simulink model "Auxiliary_Models"  (R2020b)
settings: Solver=VariableStepAuto  StartTime=0.0  StopTime=10.0  RelTol=1e-3
undefined symbols (not defined in the file or in its folder): Actuators, Ki, Klp, Klz, Kp, Kr, TestSequence, TrimPoint
libraries: simulink x19
settings Model: Creator=NicolasS  LastModifiedBy=benjaminh

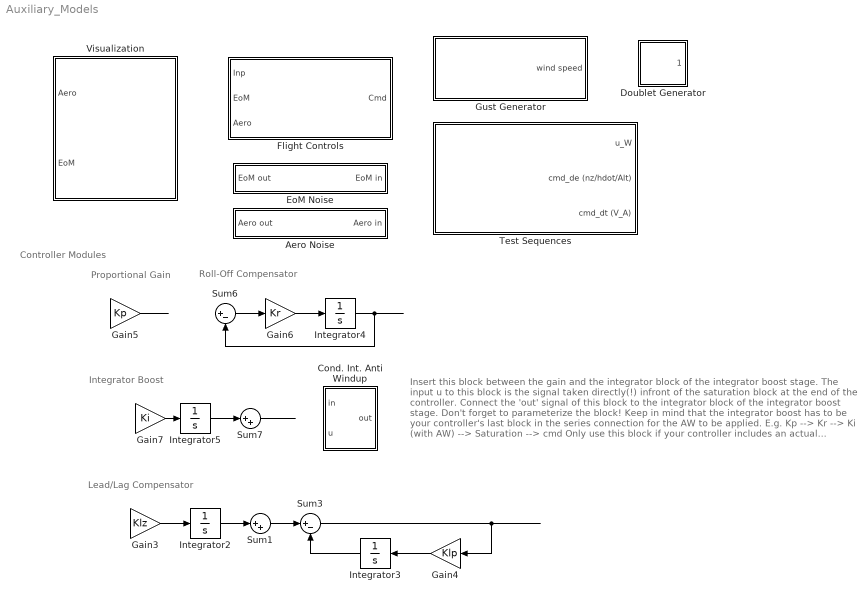
== system Auxiliary_Models ==
  note: Insert this block between the gain and the integrator block of the integrator boost stage.
      | The input u to this block is the signal taken directly(!) infront of the saturation block at the end of the controller. Connect the 'out' signal of this block to the integrator block of the integrator boost stage. Don't forget to parameterize the block!
      | Keep in mind that the integrator boost has to be your controller's last block in the series connection for the AW to be applied. E.g. Kp --> Kr --> Ki (with AW) --> Saturation --> cmd
      | Only use this block if your controller includes an actual integrator (integrator boost/pole at zero).
  note: Controller Modules
  note: Integrator Boost
  note: Roll-Off Compensator
  note: Proportional
      | Gain
  note: Lead/Lag Compensator
  Aero Noise : Subsystem
  Cond. Int. Anti Windup : Subsystem  mask(Integrator Anti-Windup){max_u=inf, min_u=-inf, negative_sign=off}
      mask prompts: max_u "Maximum control signal"; min_u "Minimum control signal"; negative_sign "Negative amplification in control law"
      mask help:
      | This block provides integration using the "conditional integration" anti-windup compensation.
      | It compares the sign of the error and the sign of the control signal and stops integration in case the error drives saturation.
      mask Help:
      | This block provides integration using the "conditional integration" anti-windup compensation. It stops or continues integration depending on the sign of the integrator input (control error) and the commanded control signal. Only if the input would further increase the already saturated integrator output, integration is stopped. This method is different from "integrator clamping" and and "integrator back calculation" and usually provides better recovery properties.
      | 
      | In a standard control architecture the inputs are as follows:
      | INPUT is the error signal r-y
      | RESET is a reset signal. The integrator state is reseted on either rising or falling edges
      | X0 is the initial condition for the integrator
      | U is the commanded control signal
      | 
      | For the anti-windup to work as intended, a saturation block must be placed on the ouput of the control command being fed to the associated actuator, which should include all control signal contributions (e.g. from proportional feedback and inner loops). U is the signal before this saturation.
      | 
      | The default logic assumes a plant with positive steady-state gain to be controlled. This translates to the following logic:
      | For commanded control signal u, saturation limits Umax and Umin, and error e,
      | If u is in bounds, do nothing
      | If u >= Umax AND e > 0, stop integrating
      | If u >= Umax AND e < 0, continue integrating
      | If u <= Umin AND e > 0, continue integrating
      | If u <= Umin AND e < 0, stop integrating
      | 
      | If a plant with negative steady-state gain is to be controlled (e.g. pitch), the windup logic may changed using the NEGATIVE SIGN option. (Note: If unsure check if the controller gains are negative. If yes, check the NEGATIVE SIGN option)
      | This then translates to the logic:
      | If u is in bounds, do nothing
      | If u >= Umax AND e < 0, stop integrating
      | If u >= Umax AND e > 0, continue integrating
      | If u <= Umin AND e < 0, continue integrating
      | If u <= Umin AND e > 0, stop integrating
  Doublet Generator : Subsystem  mask(DoubletGenerator){timeon=0, pulsewidth=1, amplitude=1}
      mask prompts: timeon "Time Start"; pulsewidth "Pulse Duration"
      mask help:
      | Doublet Generator.
      | Ouputs doublet of specificed amplitude and duration.
      |
      | If start/duration/amplitude parameters are vectors, then output is multichannel.
      mask Display: plot([.1 .3 .3001 .4 .4001 .5  .5001 .7],[0 0 1 1 -1 -1 0 0])
  EoM Noise : Subsystem
  Flight Controls : Subsystem
  Gain3 : Gain  Gain=Klz
  Gain4 : Gain  Gain=Klp
  Gain5 : Gain  Gain=Kp
  Gain6 : Gain  Gain=Kr
  Gain7 : Gain  Gain=Ki
  Gust Generator : Subsystem  mask{gust_start=0, gust_duration=0, gust_amplitude=0}
      mask prompts: gust_start "start time of the gust in sec"; gust_duration "gust duration in sec"; gust_amplitude "maximum gust speed in m/s"
      mask DialogControl ParameterGroupVar Prompt: gust characteristics
  Integrator{2..5} (4 alike) : Integrator  UpperSaturationLimit=max(Actuators.Limits.u_max_He)  LowerSaturationLimit=min(Actuators.Limits.u_max_He)  ContinuousStateAttributes='K'
  Sum1 : Sum  Inputs=|++
  Sum3 : Sum  Inputs=|+-
  Sum6 : Sum  Inputs=|+-
  Sum7 : Sum  Inputs=|++
  Test Sequences : Subsystem  InitFcn=|  StopFcn=clear TestSequence
      | if not(exist('TestSequence','var'))
      |        TestSequence = 0;
      | end
  Visualization : Subsystem
  wires:
  Sum7/1 -> ?
  Gain7/1 -> Integrator5/1
  Sum6/1 -> Gain6/1
  Integrator5/1 -> Sum7/1
  Gain6/1 -> Integrator4/1
  ? -> Gain5/1
  ? -> Gain7/1, Sum7/2
  Gain5/1 -> ?
  ? -> Sum6/1
  Integrator4/1 -> Sum6/2
  ? -> Sum1/2, Gain3/1
  Integrator2/1 -> Sum1/1
  Sum1/1 -> Sum3/1
  Gain4/1 -> Integrator3/1
  Integrator3/1 -> Sum3/2
  Sum3/1 -> Gain4/1
  Gain3/1 -> Integrator2/1

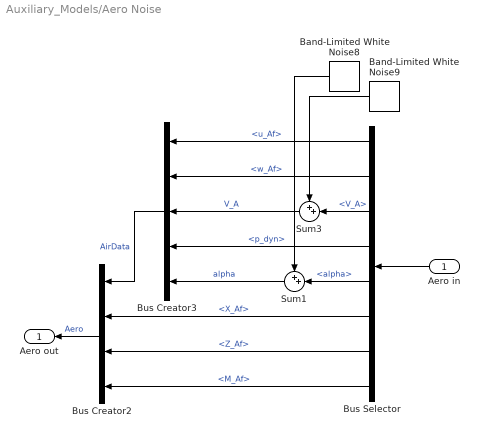
== system Auxiliary_Models/Aero Noise ==
  Aero in : Inport  OutDataTypeStr=Bus: Aero
  Band-Limited White Noise8 : simulink/Sources/Band-Limited White Noise  Cov=1E-7  Ts=0.01  seed=3324
  Band-Limited White Noise9 : simulink/Sources/Band-Limited White Noise  Cov=1E-3  Ts=0.05  seed=8153
  Bus Creator2 : BusCreator  Inputs=4  OutDataTypeStr=Bus: Aero
  Bus Creator3 : BusCreator  Inputs=5  OutDataTypeStr=Bus: AirData
  Bus Selector : BusSelector  OutputSignals=AirData.u_Af,AirData.w_Af,AirData.V_A,AirData.p_dyn,AirData.alpha,X_Af,Z_Af,M_Af
  Sum1 : Sum  Inputs=++|
  Sum3 : Sum  Inputs=++|
  Aero out : Outport  OutDataTypeStr=Bus: Aero
  wires:
  Aero in/1 -> Bus Selector/1
  Bus Creator3/1 -> Bus Creator2/1  "AirData"
  Bus Selector/6 -> Bus Creator2/2  "<X_Af>"
  Bus Selector/7 -> Bus Creator2/3  "<Z_Af>"
  Bus Selector/8 -> Bus Creator2/4  "<M_Af>"
  Bus Creator2/1 -> Aero out/1  "Aero"
  Bus Selector/1 -> Bus Creator3/1  "<u_Af>"
  Bus Selector/2 -> Bus Creator3/2  "<w_Af>"
  Bus Selector/3 -> Sum3/2  "<V_A>"
  Bus Selector/5 -> Sum1/2  "<alpha>"
  Band-Limited White Noise8/1 -> Sum1/1
  Sum1/1 -> Bus Creator3/5  "alpha"
  Bus Selector/4 -> Bus Creator3/4  "<p_dyn>"
  Band-Limited White Noise9/1 -> Sum3/1
  Sum3/1 -> Bus Creator3/3  "V_A"

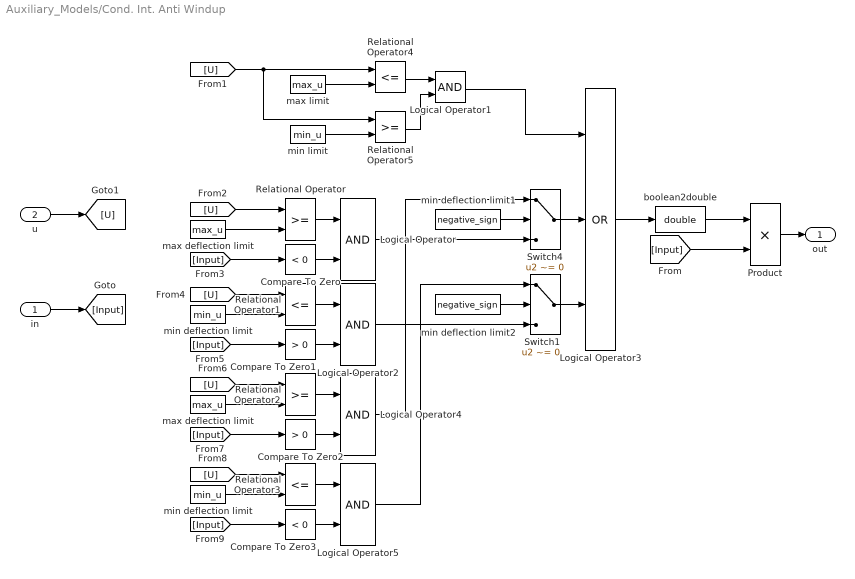
== system Auxiliary_Models/Cond. Int. Anti Windup ==
  in : Inport
  u : Inport  Port=2
  Compare To Zero : simulink/Logic and Bit Operations/Compare To Zero  relop=<  OutDataTypeStr=uint8
  Compare To Zero1 : simulink/Logic and Bit Operations/Compare To Zero  relop=>  OutDataTypeStr=uint8
  Compare To Zero2 : simulink/Logic and Bit Operations/Compare To Zero  relop=>  OutDataTypeStr=uint8
  Compare To Zero3 : simulink/Logic and Bit Operations/Compare To Zero  relop=<  OutDataTypeStr=uint8
  Logical Operator{,1..2,4..5} (5 alike) : Logic  AllPortsSameDT=off  OutDataTypeStr=boolean
  Logical Operator3 : Logic  Operator=OR  Inputs=3  AllPortsSameDT=off  OutDataTypeStr=boolean
  Product : Product
  Relational Operator : RelationalOperator  OutDataTypeStr=boolean  RndMeth=Nearest
  Relational Operator1 : RelationalOperator  Operator=<=  OutDataTypeStr=boolean  RndMeth=Nearest
  Relational Operator2 : RelationalOperator  OutDataTypeStr=boolean  RndMeth=Nearest
  Relational Operator3 : RelationalOperator  Operator=<=  OutDataTypeStr=boolean  RndMeth=Nearest
  Relational Operator4 : RelationalOperator  Operator=<=  OutDataTypeStr=boolean  RndMeth=Nearest
  Relational Operator5 : RelationalOperator  OutDataTypeStr=boolean  RndMeth=Nearest
  Switch1 : Switch  Criteria=u2 ~= 0
  Switch4 : Switch  Criteria=u2 ~= 0
  boolean2double : DataTypeConversion  OutDataTypeStr=double
  max deflection limit : Constant  Value=max_u  SampleTime=-1
  "max deflection limit " : Constant  Value=max_u  SampleTime=-1
  max limit : Constant  Value=max_u  SampleTime=-1
  min deflection limit : Constant  Value=min_u  SampleTime=-1
  "min deflection limit " : Constant  Value=min_u  SampleTime=-1
  min deflection limit1 : Constant  Value=negative_sign  SampleTime=-1
  min deflection limit2 : Constant  Value=negative_sign  SampleTime=-1
  min limit : Constant  Value=min_u  SampleTime=-1
  out : Outport
  wires:
  Product/1 -> out/1
  Logical Operator3/1 -> boolean2double/1
  boolean2double/1 -> Product/1
  [Input] -> Product/2
  [Input] -> Compare To Zero3/1
  [U] -> Relational Operator3/1
  [Input] -> Compare To Zero2/1
  [U] -> Relational Operator2/1
  [Input] -> Compare To Zero1/1
  [U] -> Relational Operator1/1
  [Input] -> Compare To Zero/1
  [U] -> Relational Operator/1
  [U] -> Relational Operator4/1, Relational Operator5/1
  u/1 -> [U]
  in/1 -> [Input]
  min limit/1 -> Relational Operator5/2
  Relational Operator5/1 -> Logical Operator1/2
  Relational Operator4/1 -> Logical Operator1/1
  max limit/1 -> Relational Operator4/2
  Logical Operator5/1 -> Switch1/1
  Logical Operator4/1 -> Switch4/1
  Logical Operator2/1 -> Switch1/3
  Logical Operator/1 -> Switch4/3
  min deflection limit1/1 -> Switch4/2
  Switch1/1 -> Logical Operator3/3
  min deflection limit2/1 -> Switch1/2
  max deflection limit/1 -> Relational Operator/2
  Compare To Zero/1 -> Logical Operator/2
  Relational Operator/1 -> Logical Operator/1
  Compare To Zero1/1 -> Logical Operator2/2
  Relational Operator1/1 -> Logical Operator2/1
  min deflection limit/1 -> Relational Operator1/2
  Switch4/1 -> Logical Operator3/2
  Logical Operator1/1 -> Logical Operator3/1
  Compare To Zero2/1 -> Logical Operator4/2
  Relational Operator2/1 -> Logical Operator4/1
  Compare To Zero3/1 -> Logical Operator5/2
  Relational Operator3/1 -> Logical Operator5/1
  "min deflection limit "/1 -> Relational Operator3/2
  "max deflection limit "/1 -> Relational Operator2/2

== system Auxiliary_Models/Doublet Generator ==
  Add : Sum  Inputs=+++
  DownStep : Step  Time=timeon+pulsewidth  After=-2  SampleTime=0
  Gain : Gain  Gain=amplitude
  UnStep : Step  Time=timeon+2*pulsewidth  SampleTime=0
  UpStep : Step  Time=timeon  SampleTime=0
  Doublet : Outport
  wires:
  UpStep/1 -> Add/1
  DownStep/1 -> Add/2
  UnStep/1 -> Add/3
  Add/1 -> Gain/1
  Gain/1 -> Doublet/1

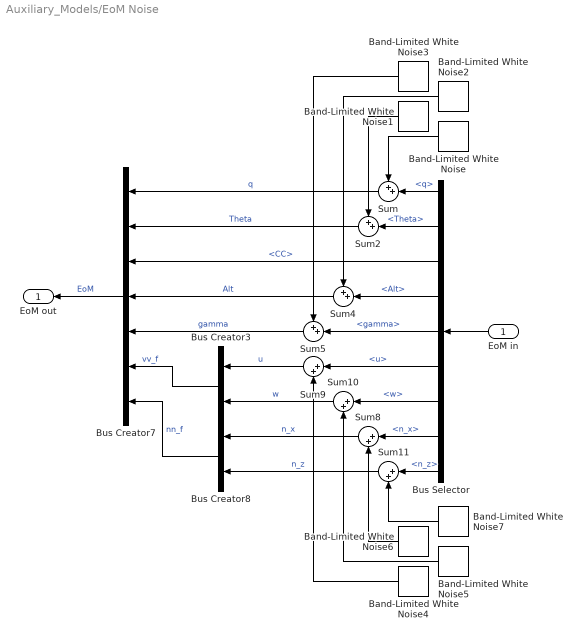
== system Auxiliary_Models/EoM Noise ==
  EoM in : Inport  OutDataTypeStr=Bus: EoM
  Band-Limited White Noise : simulink/Sources/Band-Limited White Noise  Cov=1E-5  Ts=0.01  seed=[23341]
  Band-Limited White Noise1 : simulink/Sources/Band-Limited White Noise  Cov=5E-7  Ts=0.01  seed=45875
  Band-Limited White Noise2 : simulink/Sources/Band-Limited White Noise  Cov=1E-4  Ts=0.1  seed=6874
  Band-Limited White Noise3 : simulink/Sources/Band-Limited White Noise  Cov=1E-7  Ts=0.01  seed=8153
  Band-Limited White Noise4 : simulink/Sources/Band-Limited White Noise  Cov=5E-5  Ts=0.1  seed=54769
  Band-Limited White Noise5 : simulink/Sources/Band-Limited White Noise  Cov=1E-4  Ts=0.01  seed=6932
  Band-Limited White Noise6 : simulink/Sources/Band-Limited White Noise  Cov=1E-5  Ts=0.01  seed=11452
  Band-Limited White Noise7 : simulink/Sources/Band-Limited White Noise  Cov=1E-5  Ts=0.01  seed=3324
  Bus Creator3 : BusCreator  Inputs=2  OutDataTypeStr=Bus: vv_f
  Bus Creator7 : BusCreator  Inputs=7  OutDataTypeStr=Bus: EoM
  Bus Creator8 : BusCreator  Inputs=2  OutDataTypeStr=Bus: nn_f
  Bus Selector : BusSelector  OutputSignals=q,Theta,CC,Alt,gamma,vv_f.u,vv_f.w,nn_f.n_x,nn_f.n_z
  Sum{,2,4..5} (4 alike) : Sum  Inputs=++|
  Sum{8..11} (4 alike) : Sum  Inputs=|++
  EoM out : Outport  OutDataTypeStr=Bus: EoM
  wires:
  Bus Selector/3 -> Bus Creator7/3  "<CC>"
  Bus Selector/9 -> Sum11/1  "<n_z>"
  Sum5/1 -> Bus Creator7/5  "gamma"
  Bus Creator8/1 -> Bus Creator7/7  "nn_f"
  Sum8/1 -> Bus Creator8/1  "n_x"
  Band-Limited White Noise/1 -> Sum/1
  Bus Selector/5 -> Sum5/2  "<gamma>"
  EoM in/1 -> Bus Selector/1
  Bus Selector/4 -> Sum4/2  "<Alt>"
  Bus Creator7/1 -> EoM out/1  "EoM"
  Band-Limited White Noise5/1 -> Sum10/2
  Bus Selector/8 -> Sum8/1  "<n_x>"
  Bus Creator3/1 -> Bus Creator7/6  "vv_f"
  Sum2/1 -> Bus Creator7/2  "Theta"
  Sum9/1 -> Bus Creator3/1  "u"
  Sum11/1 -> Bus Creator8/2  "n_z"
  Band-Limited White Noise3/1 -> Sum5/1
  Sum/1 -> Bus Creator7/1  "q"
  Band-Limited White Noise2/1 -> Sum4/1
  Bus Selector/6 -> Sum9/1  "<u>"
  Bus Selector/2 -> Sum2/2  "<Theta>"
  Band-Limited White Noise7/1 -> Sum11/2
  Bus Selector/7 -> Sum10/1  "<w>"
  Band-Limited White Noise4/1 -> Sum9/2
  Band-Limited White Noise1/1 -> Sum2/1
  Band-Limited White Noise6/1 -> Sum8/2
  Sum10/1 -> Bus Creator3/2  "w"
  Bus Selector/1 -> Sum/2  "<q>"
  Sum4/1 -> Bus Creator7/4  "Alt"

== system Auxiliary_Models/Flight Controls ==
  Inp : Inport
  EoM : Inport  Port=2  OutDataTypeStr=Bus: EoM
  Aero : Inport  Port=3  OutDataTypeStr=Bus: Aero
  Bus Creator2 : BusCreator  Inputs=2  OutDataTypeStr=Bus: Cmd
  Longitudinal Control Laws : Subsystem
  Cmd : Outport
  wires:
  EoM/1 -> Longitudinal Control Laws/2(EoM)
  Bus Creator2/1 -> Cmd/1  "Cmd"
  Longitudinal Control Laws/2(cmd_dt) -> Bus Creator2/2  "cmd_dt"
  Longitudinal Control Laws/1(cmd_de) -> Bus Creator2/1  "cmd_de"
  Inp/1 -> Longitudinal Control Laws/3(Inp)
  Aero/1 -> Longitudinal Control Laws/1(Aero)

== system Auxiliary_Models/Gust Generator ==
  1-cos gust : Subsystem  TreatAsAtomicUnit=on
  Clock : Clock
  Compare To Constant : simulink/Logic and Bit Operations/Compare To Constant  relop=>=  const=gust_start  OutDataTypeStr=boolean
  Constant : Constant  Value=0
  Sum : Sum  Inputs=+-|
  Switch : Switch  Criteria=u2 > Threshold  Threshold=gust_start+gust_duration
  time freeze : Subsystem  TreatAsAtomicUnit=on
  wind speed : Outport
  wires:
  time freeze/1(out) -> Sum/2
  Constant/1 -> Switch/1
  Clock/1 -> time freeze/1(in), Compare To Constant/1, Sum/1, Switch/2
  Compare To Constant/1 -> 1-cos gust/Enable, time freeze/Trigger
  Sum/1 -> 1-cos gust/1(in)
  1-cos gust/1(wind) -> Switch/3
  Switch/1 -> wind speed/1

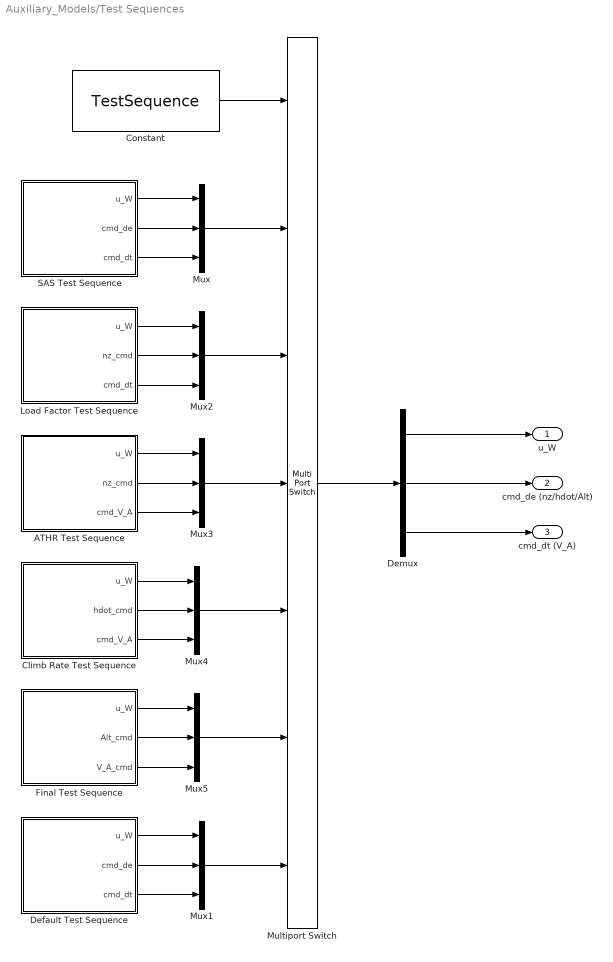
== system Auxiliary_Models/Test Sequences ==
  ATHR Test Sequence : Subsystem
  Climb Rate Test Sequence : Subsystem
  Constant : Constant  Value=TestSequence
  Default Test Sequence : Subsystem
  Demux : Demux  Outputs=3
  Final Test Sequence : Subsystem
  Load Factor Test Sequence : Subsystem
  Multiport Switch : MultiPortSwitch  Inputs=6
  Mux{,1..5} (6 alike) : Mux  Inputs=3
  SAS Test Sequence : Subsystem
  u_W : Outport
  cmd_de (nz/hdot/Alt) : Outport  Port=2
  cmd_dt (V_A) : Outport  Port=3
  wires:
  Demux/1 -> u_W/1
  Demux/2 -> cmd_de (nz/hdot/Alt)/1
  Demux/3 -> cmd_dt (V_A)/1
  Constant/1 -> Multiport Switch/1
  SAS Test Sequence/1(u_W) -> Mux/1
  SAS Test Sequence/2(cmd_de) -> Mux/2
  SAS Test Sequence/3(cmd_dt) -> Mux/3
  Mux/1 -> Multiport Switch/2
  Multiport Switch/1 -> Demux/1
  Default Test Sequence/1(u_W) -> Mux1/1
  Default Test Sequence/2(cmd_de) -> Mux1/2
  Default Test Sequence/3(cmd_dt) -> Mux1/3
  Mux1/1 -> Multiport Switch/7
  Load Factor Test Sequence/1(u_W) -> Mux2/1
  Load Factor Test Sequence/2(nz_cmd) -> Mux2/2
  Load Factor Test Sequence/3(cmd_dt) -> Mux2/3
  Mux2/1 -> Multiport Switch/3
  ATHR Test Sequence/1(u_W) -> Mux3/1
  ATHR Test Sequence/2(nz_cmd) -> Mux3/2
  ATHR Test Sequence/3(cmd_V_A) -> Mux3/3
  Mux3/1 -> Multiport Switch/4
  Climb Rate Test Sequence/1(u_W) -> Mux4/1
  Climb Rate Test Sequence/2(hdot_cmd) -> Mux4/2
  Climb Rate Test Sequence/3(cmd_V_A) -> Mux4/3
  Mux4/1 -> Multiport Switch/5
  Final Test Sequence/1(u_W) -> Mux5/1
  Final Test Sequence/2(Alt_cmd) -> Mux5/2
  Final Test Sequence/3(V_A_cmd) -> Mux5/3
  Mux5/1 -> Multiport Switch/6

== system Auxiliary_Models/Visualization ==
  Aero : Inport  OutDataTypeStr=Bus: Aero
  EoM : Inport  Port=2  OutDataTypeStr=Bus: EoM
  Bus Selector2 : BusSelector  OutputSignals=OOmega_f.q,vv_f.u,vv_f.w,PPhi.Theta,Position.Alt,nn_f.n_z
  Bus Selector3 : BusSelector  OutputSignals=AirData.alpha
  Gain11 : Gain  Gain=180/pi
  Gain8 : Gain  Gain=180/pi
  Gain9 : Gain  Gain=180/pi
  Scope2 : Scope  NumInputPorts=7
  wires:
  Gain8/1 -> Scope2/2  "q"
  Gain11/1 -> Scope2/1  "alpha"
  Gain9/1 -> Scope2/5  "Theta"
  Aero/1 -> Bus Selector3/1
  Bus Selector2/2 -> Scope2/3  "<u>"
  Bus Selector2/1 -> Gain8/1  "<q>"
  EoM/1 -> Bus Selector2/1
  Bus Selector2/6 -> Scope2/7  "<n_z>"
  Bus Selector2/5 -> Scope2/6  "<Alt>"
  Bus Selector3/1 -> Gain11/1  "<alpha>"
  Bus Selector2/3 -> Scope2/4  "<w>"
  Bus Selector2/4 -> Gain9/1  "<Theta>"

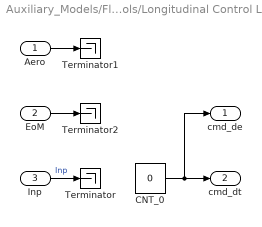
== system Auxiliary_Models/Flight Controls/Longitudinal Control Laws ==
  Aero : Inport  OutDataTypeStr=Bus: Aero
  EoM : Inport  Port=2  OutDataTypeStr=Bus: EoM
  Inp : Inport  Port=3
  CNT_0 : Constant  Value=0
  Terminator : Terminator
  Terminator1 : Terminator
  Terminator2 : Terminator
  cmd_de : Outport
  cmd_dt : Outport  Port=2
  wires:
  CNT_0/1 -> cmd_de/1, cmd_dt/1
  Inp/1 -> Terminator/1  "Inp"
  Aero/1 -> Terminator1/1
  EoM/1 -> Terminator2/1

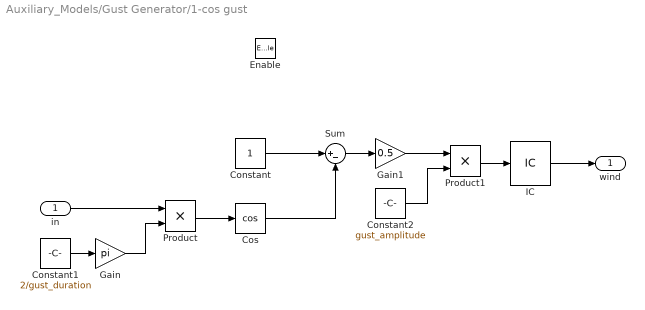
== system Auxiliary_Models/Gust Generator/1-cos gust ==
  in : Inport
  Enable : EnablePort  StatesWhenEnabling=reset
  Constant : Constant
  Constant1 : Constant  Value=2/gust_duration
  Constant2 : Constant  Value=gust_amplitude
  Cos : Trigonometry  Operator=cos
  Gain : Gain  Gain=pi
  Gain1 : Gain  Gain=0.5
  IC : InitialCondition  Value=0
  Product : Product
  Product1 : Product
  Sum : Sum  Inputs=|+-
  wind : Outport
  wires:
  IC/1 -> wind/1
  Constant1/1 -> Gain/1
  Product1/1 -> IC/1
  Product/1 -> Cos/1
  Cos/1 -> Sum/2
  Constant/1 -> Sum/1
  Gain/1 -> Product/2
  Gain1/1 -> Product1/1
  Sum/1 -> Gain1/1
  Constant2/1 -> Product1/2
  in/1 -> Product/1

== system Auxiliary_Models/Gust Generator/time freeze ==
  in : Inport
  Trigger : TriggerPort  VariantControl=Variant
  out : Outport  InitialOutput=0
  wires:
  in/1 -> out/1

== system Auxiliary_Models/Test Sequences/ATHR Test Sequence ==
  Add : Sum
  Constant1 : Constant  Value=0
  Constant2 : Constant  Value=sqrt(TrimPoint.States.ubar^2+TrimPoint.States.wbar^2)
  Doublet Generator : Subsystem  mask(DoubletGenerator){timeon=5, pulsewidth=30, amplitude=10}
      mask prompts: timeon "Time Start"; pulsewidth "Pulse Duration"
      mask help:
      | Doublet Generator.
      | Ouputs doublet of specificed amplitude and duration.
      |
      | If start/duration/amplitude parameters are vectors, then output is multichannel.
      mask Display: plot([.1 .3 .3001 .4 .4001 .5  .5001 .7],[0 0 1 1 -1 -1 0 0])
  Gust Generator : Subsystem  mask{gust_start=100, gust_duration=15, gust_amplitude=20}
      mask prompts: gust_start "start time of the gust in sec"; gust_duration "gust duration in sec"; gust_amplitude "maximum gust speed in m/s"
      mask DialogControl ParameterGroupVar Prompt: gust characteristics
  u_W : Outport  PortDimensions=1
  nz_cmd : Outport  Port=2
  cmd_V_A : Outport  Port=3
  wires:
  Constant1/1 -> nz_cmd/1  "nz_cmd"
  Doublet Generator/1(Doublet) -> Add/1
  Gust Generator/1(wind speed) -> u_W/1  "u_W"
  Add/1 -> cmd_V_A/1  "cmd_V_A"
  Constant2/1 -> Add/2  "nz_cmd"

== system Auxiliary_Models/Test Sequences/Climb Rate Test Sequence ==
  Constant1 : Constant  Value=0
  Constant2 : Constant  Value=sqrt(TrimPoint.States.ubar^2+TrimPoint.States.wbar^2)
  Doublet Generator : Subsystem  mask(DoubletGenerator){timeon=5, pulsewidth=20, amplitude=5}
      mask prompts: timeon "Time Start"; pulsewidth "Pulse Duration"
      mask help:
      | Doublet Generator.
      | Ouputs doublet of specificed amplitude and duration.
      |
      | If start/duration/amplitude parameters are vectors, then output is multichannel.
      mask Display: plot([.1 .3 .3001 .4 .4001 .5  .5001 .7],[0 0 1 1 -1 -1 0 0])
  u_W : Outport  PortDimensions=1
  hdot_cmd : Outport  Port=2
  cmd_V_A : Outport  Port=3
  wires:
  Doublet Generator/1(Doublet) -> hdot_cmd/1  "hdot_cmd"
  Constant1/1 -> u_W/1  "u_W"
  Constant2/1 -> cmd_V_A/1  "cmd_V_A"

== system Auxiliary_Models/Test Sequences/Default Test Sequence ==
  Constant : Constant  Value=TrimPoint.States.debar
  Constant1 : Constant  Value=0
  Constant2 : Constant  Value=TrimPoint.States.dtbar
  u_W : Outport  PortDimensions=1
  cmd_de : Outport  Port=2
  cmd_dt : Outport  Port=3
  wires:
  Constant/1 -> cmd_de/1  "cmd_de"
  Constant2/1 -> cmd_dt/1  "cmd_dt"
  Constant1/1 -> u_W/1  "u_W"

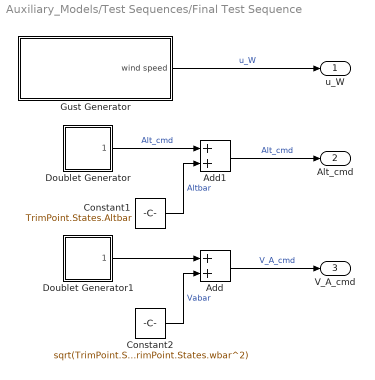
== system Auxiliary_Models/Test Sequences/Final Test Sequence ==
  Add : Sum
  Add1 : Sum
  Constant1 : Constant  Value=TrimPoint.States.Altbar
  Constant2 : Constant  Value=sqrt(TrimPoint.States.ubar^2+TrimPoint.States.wbar^2)
  Doublet Generator : Subsystem  mask(DoubletGenerator){timeon=5, pulsewidth=40, amplitude=100}
      mask prompts: timeon "Time Start"; pulsewidth "Pulse Duration"
      mask help:
      | Doublet Generator.
      | Ouputs doublet of specificed amplitude and duration.
      |
      | If start/duration/amplitude parameters are vectors, then output is multichannel.
      mask Display: plot([.1 .3 .3001 .4 .4001 .5  .5001 .7],[0 0 1 1 -1 -1 0 0])
  Doublet Generator1 : Subsystem  mask(DoubletGenerator){timeon=5, pulsewidth=60, amplitude=10}
      mask prompts: timeon "Time Start"; pulsewidth "Pulse Duration"
      mask help:
      | Doublet Generator.
      | Ouputs doublet of specificed amplitude and duration.
      |
      | If start/duration/amplitude parameters are vectors, then output is multichannel.
      mask Display: plot([.1 .3 .3001 .4 .4001 .5  .5001 .7],[0 0 1 1 -1 -1 0 0])
  Gust Generator : Subsystem  mask{gust_start=30, gust_duration=15, gust_amplitude=20}
      mask prompts: gust_start "start time of the gust in sec"; gust_duration "gust duration in sec"; gust_amplitude "maximum gust speed in m/s"
      mask DialogControl ParameterGroupVar Prompt: gust characteristics
  u_W : Outport  PortDimensions=1
  Alt_cmd : Outport  Port=2
  V_A_cmd : Outport  Port=3
  wires:
  Doublet Generator/1(Doublet) -> Add1/1  "Alt_cmd"
  Gust Generator/1(wind speed) -> u_W/1  "u_W"
  Add/1 -> V_A_cmd/1  "V_A_cmd"
  Doublet Generator1/1(Doublet) -> Add/1
  Constant2/1 -> Add/2  "Vabar"
  Constant1/1 -> Add1/2  "Altbar"
  Add1/1 -> Alt_cmd/1  "Alt_cmd"

== system Auxiliary_Models/Test Sequences/Load Factor Test Sequence ==
  Constant2 : Constant  Value=TrimPoint.States.dtbar
  Doublet Generator : Subsystem  mask(DoubletGenerator){timeon=5, pulsewidth=6, amplitude=0.2}
      mask prompts: timeon "Time Start"; pulsewidth "Pulse Duration"
      mask help:
      | Doublet Generator.
      | Ouputs doublet of specificed amplitude and duration.
      |
      | If start/duration/amplitude parameters are vectors, then output is multichannel.
      mask Display: plot([.1 .3 .3001 .4 .4001 .5  .5001 .7],[0 0 1 1 -1 -1 0 0])
  Gust Generator : Subsystem  mask{gust_start=20, gust_duration=15, gust_amplitude=20}
      mask prompts: gust_start "start time of the gust in sec"; gust_duration "gust duration in sec"; gust_amplitude "maximum gust speed in m/s"
      mask DialogControl ParameterGroupVar Prompt: gust characteristics
  u_W : Outport  PortDimensions=1
  nz_cmd : Outport  Port=2
  cmd_dt : Outport  Port=3
  wires:
  Doublet Generator/1(Doublet) -> nz_cmd/1  "nz_cmd"
  Constant2/1 -> cmd_dt/1  "cmd_dt"
  Gust Generator/1(wind speed) -> u_W/1  "u_W"

== system Auxiliary_Models/Test Sequences/SAS Test Sequence ==
  Constant2 : Constant  Value=TrimPoint.States.dtbar
  Gust Generator : Subsystem  mask{gust_start=15, gust_duration=15, gust_amplitude=20}
      mask prompts: gust_start "start time of the gust in sec"; gust_duration "gust duration in sec"; gust_amplitude "maximum gust speed in m/s"
      mask DialogControl ParameterGroupVar Prompt: gust characteristics
  Step : Step  Time=5  Before=TrimPoint.States.debar  After=TrimPoint.States.debar + deg2rad(-1)  SampleTime=0
  u_W : Outport  PortDimensions=1
  cmd_de : Outport  Port=2
  cmd_dt : Outport  Port=3
  wires:
  Step/1 -> cmd_de/1  "cmd_de"
  Constant2/1 -> cmd_dt/1  "cmd_dt"
  Gust Generator/1(wind speed) -> u_W/1  "u_W"

== system Auxiliary_Models/Test Sequences/ATHR Test Sequence/Doublet Generator ==
  Add : Sum  Inputs=+++
  DownStep : Step  Time=timeon+pulsewidth  After=-1  SampleTime=0
  Gain : Gain  Gain=amplitude
  UnStep : Step  Time=timeon+2*pulsewidth  After=-1  SampleTime=0
  UpStep : Step  Time=timeon  SampleTime=0
  Doublet : Outport
  wires:
  UpStep/1 -> Add/1
  DownStep/1 -> Add/2
  UnStep/1 -> Add/3
  Add/1 -> Gain/1
  Gain/1 -> Doublet/1

== system Auxiliary_Models/Test Sequences/ATHR Test Sequence/Gust Generator ==
  1-cos gust : Subsystem  TreatAsAtomicUnit=on
  Clock : Clock
  Compare To Constant : simulink/Logic and Bit Operations/Compare To Constant  relop=>=  const=gust_start  OutDataTypeStr=boolean
  Constant : Constant  Value=0
  Sum : Sum  Inputs=+-|
  Switch : Switch  Criteria=u2 > Threshold  Threshold=gust_start+gust_duration
  time freeze : Subsystem  TreatAsAtomicUnit=on
  wind speed : Outport
  wires:
  time freeze/1(out) -> Sum/2
  Constant/1 -> Switch/1
  Clock/1 -> time freeze/1(in), Compare To Constant/1, Sum/1, Switch/2
  Compare To Constant/1 -> 1-cos gust/Enable, time freeze/Trigger
  Sum/1 -> 1-cos gust/1(in)
  1-cos gust/1(wind) -> Switch/3
  Switch/1 -> wind speed/1

== system Auxiliary_Models/Test Sequences/Climb Rate Test Sequence/Doublet Generator ==
  Add : Sum  Inputs=+++
  DownStep : Step  Time=timeon+pulsewidth  After=-2  SampleTime=0
  Gain : Gain  Gain=amplitude
  UnStep : Step  Time=timeon+2*pulsewidth  SampleTime=0
  UpStep : Step  Time=timeon  SampleTime=0
  Doublet : Outport
  wires:
  UpStep/1 -> Add/1
  DownStep/1 -> Add/2
  UnStep/1 -> Add/3
  Add/1 -> Gain/1
  Gain/1 -> Doublet/1

== system Auxiliary_Models/Test Sequences/Final Test Sequence/Doublet Generator ==
  Add : Sum  Inputs=+++
  DownStep : Step  Time=timeon+pulsewidth  After=-2  SampleTime=0
  Gain : Gain  Gain=amplitude
  UnStep : Step  Time=timeon+2*pulsewidth  SampleTime=0
  UpStep : Step  Time=timeon  SampleTime=0
  Doublet : Outport
  wires:
  UpStep/1 -> Add/1
  DownStep/1 -> Add/2
  UnStep/1 -> Add/3
  Add/1 -> Gain/1
  Gain/1 -> Doublet/1

== system Auxiliary_Models/Test Sequences/Final Test Sequence/Doublet Generator1 ==
  Add : Sum  Inputs=+++
  DownStep : Step  Time=timeon+pulsewidth  SampleTime=0
  Gain : Gain  Gain=amplitude
  UnStep : Step  Time=timeon+2*pulsewidth  After=-1  SampleTime=0
  UpStep : Step  Time=timeon  SampleTime=0
  Doublet : Outport
  wires:
  UpStep/1 -> Add/1
  DownStep/1 -> Add/2
  UnStep/1 -> Add/3
  Add/1 -> Gain/1
  Gain/1 -> Doublet/1

== system Auxiliary_Models/Test Sequences/Final Test Sequence/Gust Generator ==
  1-cos gust : Subsystem  TreatAsAtomicUnit=on
  Clock : Clock
  Compare To Constant : simulink/Logic and Bit Operations/Compare To Constant  relop=>=  const=gust_start  OutDataTypeStr=boolean
  Constant : Constant  Value=0
  Sum : Sum  Inputs=+-|
  Switch : Switch  Criteria=u2 > Threshold  Threshold=gust_start+gust_duration
  time freeze : Subsystem  TreatAsAtomicUnit=on
  wind speed : Outport
  wires:
  time freeze/1(out) -> Sum/2
  Constant/1 -> Switch/1
  Clock/1 -> time freeze/1(in), Compare To Constant/1, Sum/1, Switch/2
  Compare To Constant/1 -> 1-cos gust/Enable, time freeze/Trigger
  Sum/1 -> 1-cos gust/1(in)
  1-cos gust/1(wind) -> Switch/3
  Switch/1 -> wind speed/1

== system Auxiliary_Models/Test Sequences/Load Factor Test Sequence/Doublet Generator ==
  Add : Sum  Inputs=+++
  DownStep : Step  Time=timeon+pulsewidth  After=-2  SampleTime=0
  Gain : Gain  Gain=amplitude
  UnStep : Step  Time=timeon+2*pulsewidth  SampleTime=0
  UpStep : Step  Time=timeon  SampleTime=0
  Doublet : Outport
  wires:
  UpStep/1 -> Add/1
  DownStep/1 -> Add/2
  UnStep/1 -> Add/3
  Add/1 -> Gain/1
  Gain/1 -> Doublet/1

== system Auxiliary_Models/Test Sequences/Load Factor Test Sequence/Gust Generator ==
  1-cos gust : Subsystem  TreatAsAtomicUnit=on
  Clock : Clock
  Compare To Constant : simulink/Logic and Bit Operations/Compare To Constant  relop=>=  const=gust_start  OutDataTypeStr=boolean
  Constant : Constant  Value=0
  Sum : Sum  Inputs=+-|
  Switch : Switch  Criteria=u2 > Threshold  Threshold=gust_start+gust_duration
  time freeze : Subsystem  TreatAsAtomicUnit=on
  wind speed : Outport
  wires:
  time freeze/1(out) -> Sum/2
  Constant/1 -> Switch/1
  Clock/1 -> time freeze/1(in), Compare To Constant/1, Sum/1, Switch/2
  Compare To Constant/1 -> 1-cos gust/Enable, time freeze/Trigger
  Sum/1 -> 1-cos gust/1(in)
  1-cos gust/1(wind) -> Switch/3
  Switch/1 -> wind speed/1

== system Auxiliary_Models/Test Sequences/SAS Test Sequence/Gust Generator ==
  1-cos gust : Subsystem  TreatAsAtomicUnit=on
  Clock : Clock
  Compare To Constant : simulink/Logic and Bit Operations/Compare To Constant  relop=>=  const=gust_start  OutDataTypeStr=boolean
  Constant : Constant  Value=0
  Sum : Sum  Inputs=+-|
  Switch : Switch  Criteria=u2 > Threshold  Threshold=gust_start+gust_duration
  time freeze : Subsystem  TreatAsAtomicUnit=on
  wind speed : Outport
  wires:
  time freeze/1(out) -> Sum/2
  Constant/1 -> Switch/1
  Clock/1 -> time freeze/1(in), Compare To Constant/1, Sum/1, Switch/2
  Compare To Constant/1 -> 1-cos gust/Enable, time freeze/Trigger
  Sum/1 -> 1-cos gust/1(in)
  1-cos gust/1(wind) -> Switch/3
  Switch/1 -> wind speed/1

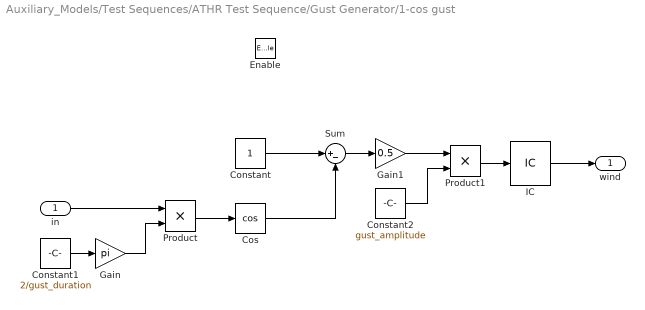
== system Auxiliary_Models/Test Sequences/ATHR Test Sequence/Gust Generator/1-cos gust ==
  in : Inport
  Enable : EnablePort  StatesWhenEnabling=reset
  Constant : Constant
  Constant1 : Constant  Value=2/gust_duration
  Constant2 : Constant  Value=gust_amplitude
  Cos : Trigonometry  Operator=cos
  Gain : Gain  Gain=pi
  Gain1 : Gain  Gain=0.5
  IC : InitialCondition  Value=0
  Product : Product
  Product1 : Product
  Sum : Sum  Inputs=|+-
  wind : Outport
  wires:
  IC/1 -> wind/1
  Constant1/1 -> Gain/1
  Product1/1 -> IC/1
  Product/1 -> Cos/1
  Cos/1 -> Sum/2
  Constant/1 -> Sum/1
  Gain/1 -> Product/2
  Gain1/1 -> Product1/1
  Sum/1 -> Gain1/1
  Constant2/1 -> Product1/2
  in/1 -> Product/1

== system Auxiliary_Models/Test Sequences/ATHR Test Sequence/Gust Generator/time freeze ==
  in : Inport
  Trigger : TriggerPort  VariantControl=Variant
  out : Outport  InitialOutput=0
  wires:
  in/1 -> out/1

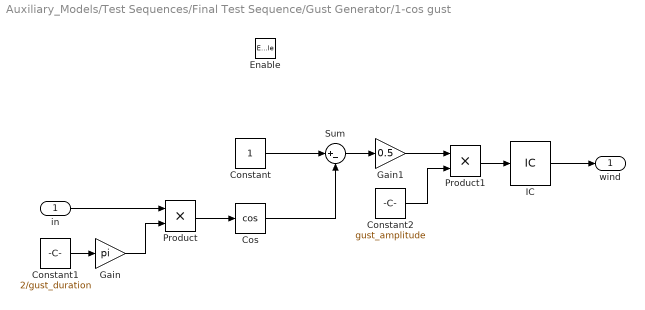
== system Auxiliary_Models/Test Sequences/Final Test Sequence/Gust Generator/1-cos gust ==
  in : Inport
  Enable : EnablePort  StatesWhenEnabling=reset
  Constant : Constant
  Constant1 : Constant  Value=2/gust_duration
  Constant2 : Constant  Value=gust_amplitude
  Cos : Trigonometry  Operator=cos
  Gain : Gain  Gain=pi
  Gain1 : Gain  Gain=0.5
  IC : InitialCondition  Value=0
  Product : Product
  Product1 : Product
  Sum : Sum  Inputs=|+-
  wind : Outport
  wires:
  IC/1 -> wind/1
  Constant1/1 -> Gain/1
  Product1/1 -> IC/1
  Product/1 -> Cos/1
  Cos/1 -> Sum/2
  Constant/1 -> Sum/1
  Gain/1 -> Product/2
  Gain1/1 -> Product1/1
  Sum/1 -> Gain1/1
  Constant2/1 -> Product1/2
  in/1 -> Product/1

== system Auxiliary_Models/Test Sequences/Final Test Sequence/Gust Generator/time freeze ==
  in : Inport
  Trigger : TriggerPort  VariantControl=Variant
  out : Outport  InitialOutput=0
  wires:
  in/1 -> out/1

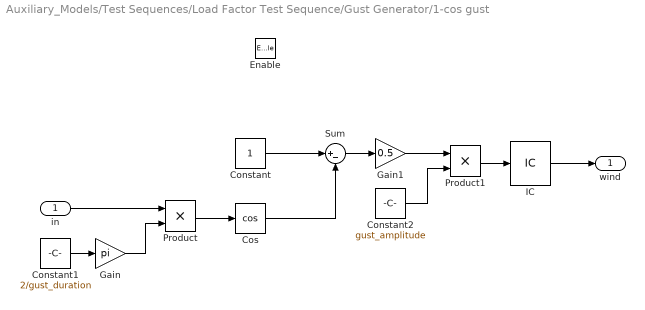
== system Auxiliary_Models/Test Sequences/Load Factor Test Sequence/Gust Generator/1-cos gust ==
  in : Inport
  Enable : EnablePort  StatesWhenEnabling=reset
  Constant : Constant
  Constant1 : Constant  Value=2/gust_duration
  Constant2 : Constant  Value=gust_amplitude
  Cos : Trigonometry  Operator=cos
  Gain : Gain  Gain=pi
  Gain1 : Gain  Gain=0.5
  IC : InitialCondition  Value=0
  Product : Product
  Product1 : Product
  Sum : Sum  Inputs=|+-
  wind : Outport
  wires:
  IC/1 -> wind/1
  Constant1/1 -> Gain/1
  Product1/1 -> IC/1
  Product/1 -> Cos/1
  Cos/1 -> Sum/2
  Constant/1 -> Sum/1
  Gain/1 -> Product/2
  Gain1/1 -> Product1/1
  Sum/1 -> Gain1/1
  Constant2/1 -> Product1/2
  in/1 -> Product/1

== system Auxiliary_Models/Test Sequences/Load Factor Test Sequence/Gust Generator/time freeze ==
  in : Inport
  Trigger : TriggerPort  VariantControl=Variant
  out : Outport  InitialOutput=0
  wires:
  in/1 -> out/1

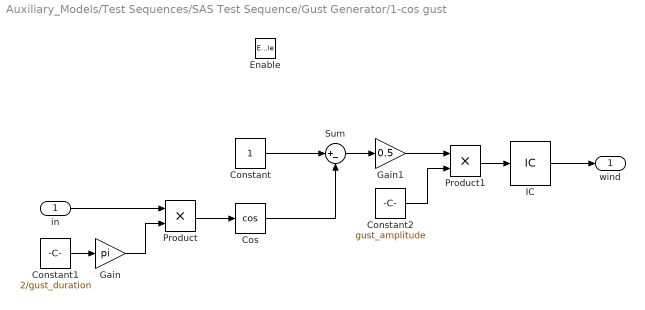
== system Auxiliary_Models/Test Sequences/SAS Test Sequence/Gust Generator/1-cos gust ==
  in : Inport
  Enable : EnablePort  StatesWhenEnabling=reset
  Constant : Constant
  Constant1 : Constant  Value=2/gust_duration
  Constant2 : Constant  Value=gust_amplitude
  Cos : Trigonometry  Operator=cos
  Gain : Gain  Gain=pi
  Gain1 : Gain  Gain=0.5
  IC : InitialCondition  Value=0
  Product : Product
  Product1 : Product
  Sum : Sum  Inputs=|+-
  wind : Outport
  wires:
  IC/1 -> wind/1
  Constant1/1 -> Gain/1
  Product1/1 -> IC/1
  Product/1 -> Cos/1
  Cos/1 -> Sum/2
  Constant/1 -> Sum/1
  Gain/1 -> Product/2
  Gain1/1 -> Product1/1
  Sum/1 -> Gain1/1
  Constant2/1 -> Product1/2
  in/1 -> Product/1

== system Auxiliary_Models/Test Sequences/SAS Test Sequence/Gust Generator/time freeze ==
  in : Inport
  Trigger : TriggerPort  VariantControl=Variant
  out : Outport  InitialOutput=0
  wires:
  in/1 -> out/1
